simulink model "bh_proto_swingup_NEGATE_DAMPING"  (R2017a)
settings: Solver=ode4  StartTime=0.0  StopTime=11  FixedStep=0.001  RelTol=1e-5  EnableMultiTasking=on
values from neighbouring files (symbols this model uses):
  b3_damp = res_T.b3_damp    [bh_pend_solve_ODE_sys.m]
  Io3_xx = res_T.Io3_xx    [bh_pend_solve_ODE_sys.m]
  L3y = res_T.L3y    [bh_pend_solve_ODE_sys.m]    (also in bh_pend_solve_ODE_sys_custom.m)
  m = res_T.mass3    [bh_pend_solve_ODE_sys_custom.m]
  mass3 = res_T.mass3    [bh_pend_solve_ODE_sys.m]    (also in bh_pend_solve_ODE_sys_custom.m)
  N = 1 + N_steps    [bh_pend_solve_ODE_sys_custom.m]
undefined symbols (not defined in the file or in its folder): L3x, L3z, X, Y, Z
libraries: sm_lib x12, simulink_extras x11, nesl_utility x8, simulink x2
settings Model: Creator=bhorton  LastModifiedBy=bhorton
settings SolverCC: ZeroCrossAlgorithm=Adaptive
settings OptimizationCC: LifeSpan=inf
settings DebuggingCC: SFUnexpectedBacktrackingDiag=warning  SFNoUnconditionalDefaultTransitionDiag=warning  SFExecutionAtInitializationDiag=none
settings GRTTargetCC: TargetLangStandard=C89/C90 (ANSI)
settings ConfigComp: CovMetricSettings=dw  CovHtmlReporting=on  CovSaveCumulativeToWorkspaceVar=on  CovSaveSingleToWorkspaceVar=on  CovExternalEMLEnable=off
settings SimscapeCC: SimscapeLogType=all  SimscapeLogDataHistory=10000  SelectedTab=Simscape Multibody

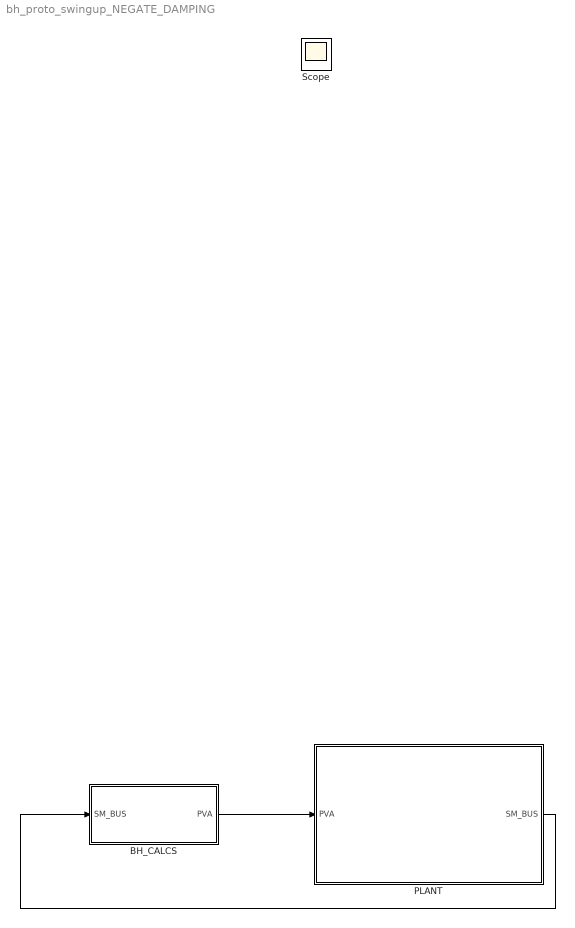
== system bh_proto_swingup_NEGATE_DAMPING ==
  BH_CALCS : Subsystem
  PLANT : Subsystem
  Scope : Scope
  wires:
  PLANT/1(SM_BUS) -> BH_CALCS/1(SM_BUS)
  BH_CALCS/1(PVA) -> PLANT/1(PVA)

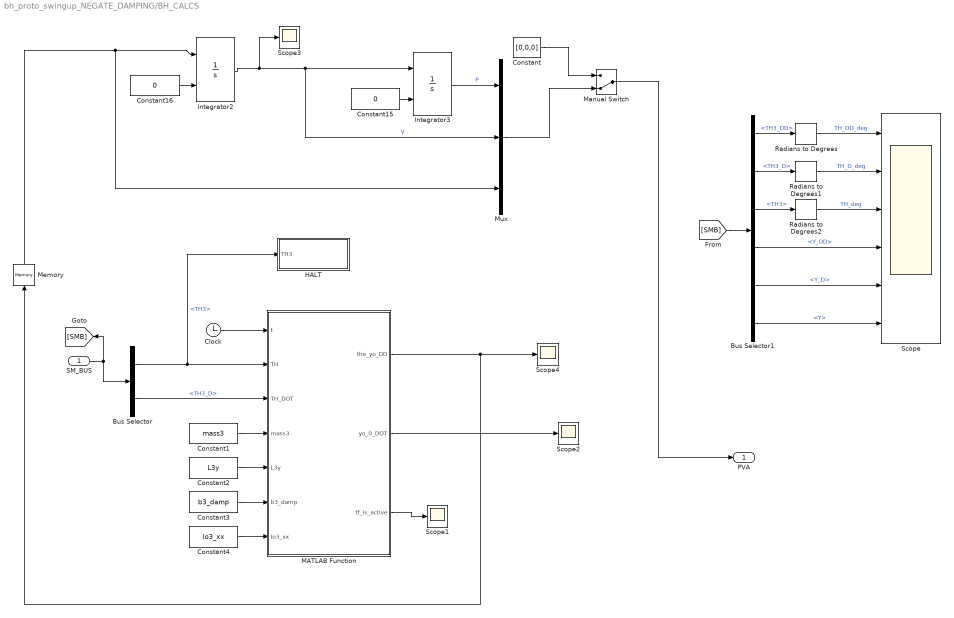
== system bh_proto_swingup_NEGATE_DAMPING/BH_CALCS ==
  SM_BUS : Inport
  Bus Selector : BusSelector  OutputSignals=TH3,TH3_D
  Bus Selector1 : BusSelector  OutputSignals=TH3_DD,TH3_D,TH3,Y_DD,Y_D,Y
  Clock : Clock
  Constant : Constant  Value=[0,0,0]
  Constant1 : Constant  Value=mass3
  Constant15 : Constant  Value=0
  Constant16 : Constant  Value=0
  Constant2 : Constant  Value=L3y
  Constant3 : Constant  Value=b3_damp
  Constant4 : Constant  Value=Io3_xx
  HALT : Subsystem
  Integrator2 : Integrator  InitialConditionSource=external
  Integrator3 : Integrator  InitialConditionSource=external
  MATLAB Function : MATLAB Function  TreatAsAtomicUnit=on  SystemSampleTime=0.001
  Manual Switch : ManualSwitch  CurrentSetting=0
  Memory : Memory
  Mux : Mux  Inputs=3
  Radians to Degrees : simulink_extras/Transformations/Radians to Degrees
  Radians to Degrees1 : simulink_extras/Transformations/Radians to Degrees
  Radians to Degrees2 : simulink_extras/Transformations/Radians to Degrees
  Scope : Scope  NumInputPorts=6
  Scope{1..4} (4 alike) : Scope
  PVA : Outport
  wires:
  Integrator3/1 -> Mux/1  "P"
  Integrator2/1 -> Scope3/1, Mux/2, Integrator3/1  "V"
  Constant15/1 -> Integrator3/2
  Manual Switch/1 -> PVA/1
  SM_BUS/1 -> [SMB], Bus Selector/1
  Bus Selector/1 -> HALT/1(TH3), MATLAB Function/2(TH)  "<TH3>"
  Bus Selector/2 -> MATLAB Function/3(TH_DOT)  "<TH3_D>"
  Memory/1 -> Mux/3, Integrator2/1
  Constant3/1 -> MATLAB Function/6(b3_damp)
  Constant2/1 -> MATLAB Function/5(L3y)
  Constant1/1 -> MATLAB Function/4(mass3)
  MATLAB Function/1(the_yo_DD) -> Scope4/1, Memory/1
  [SMB] -> Bus Selector1/1
  Bus Selector1/1 -> Radians to Degrees/1  "<TH3_DD>"
  Bus Selector1/2 -> Radians to Degrees1/1  "<TH3_D>"
  Bus Selector1/3 -> Radians to Degrees2/1  "<TH3>"
  Radians to Degrees/1 -> Scope/1  "TH_DD_deg"
  Radians to Degrees1/1 -> Scope/2  "TH_D_deg"
  Radians to Degrees2/1 -> Scope/3  "TH_deg"
  Bus Selector1/4 -> Scope/4  "<Y_DD>"
  Bus Selector1/5 -> Scope/5  "<Y_D>"
  Bus Selector1/6 -> Scope/6  "<Y>"
  Mux/1 -> Manual Switch/2
  Constant/1 -> Manual Switch/1
  Clock/1 -> MATLAB Function/1(t)
  MATLAB Function/3(tf_is_active) -> Scope1/1
  MATLAB Function/2(yo_0_DOT) -> Scope2/1
  Constant4/1 -> MATLAB Function/7(Io3_xx)
  Constant16/1 -> Integrator2/2

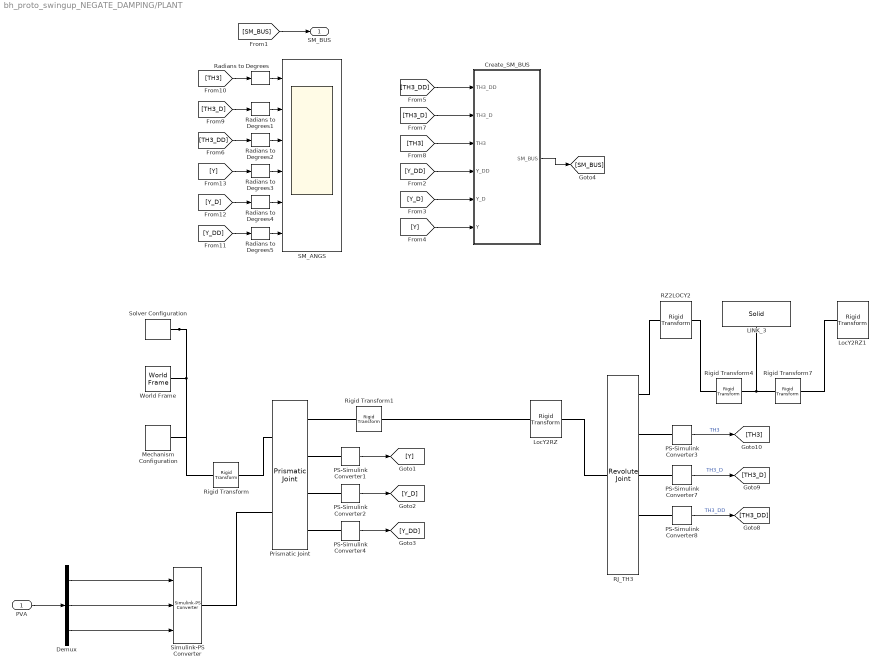
== system bh_proto_swingup_NEGATE_DAMPING/PLANT ==
  PVA : Inport
  Create_SM_BUS : Subsystem
  Demux : Demux  Outputs=3
  LINK_3 : sm_lib/Body Elements/Solid  InertiaType=CalculateFromGeometry  Mass=1  MassUnits=kg  CenterOfMass=[0 0 0]  CenterOfMassUnits=m  MomentsOfInertia=[1 1 1]  MomentsOfInertiaUnits=kg*m^2  ProductsOfInertia=[0 0 0]  ProductsOfInertiaUnits=kg*m^2  DensityBased=on  Density=density  DensityUnits=kg/(m^3)  DoExposeReferenceFrame=on  SerializedFrames=<Frames/>  GraphicType=FromGeometry  MarkerShape=Sphere  MarkerSize=10  GraphicVisPropType=SimpleVisualProperties  GraphicDiffuseColor=[1.0 0.8 0.4]  GraphicSpecularColor=[0.5 0.5 0.5 1.0]  GraphicAmbientColor=[0.15 0.15 0.15 1.0]  GraphicEmissiveColor=[0.0 0.0 0.0 1.0]  GraphicShininess=75  GraphicOpacity=1.0  GeometryShape=Brick  RectangleSize=[1 1]  RectangleSizeUnits=m  BrickDimensions=[L3x, L3y, L3z ]  BrickDimensionUnits=m  CylinderRadius=1  CylinderRadiusUnits=m  CylinderLength=1  CylinderLengthUnits=m  SphereRadius=1  SphereRadiusUnits=m  EllipsoidRadii=[1 1 1]  EllipsoidRadiiUnits=m  ExtrusionCrossSection=[1 1; -1 1; -1 -1; 1 -1]  ExtrusionCrossSectionUnits=m  ExtrusionLength=1  ExtrusionLengthUnits=m  PolygonNumSides=3  PolygonOuterRadius=1  PolygonOuterRadiusUnits=m  ExtGeomFileType=STEP  ExtGeomFileUnits=m  RevolutionCrossSection=[1 1; 1 -1; 2 -1; 2 1]  RevolutionCrossSectionUnits=m  RevolutionExtent=Full  RevolutionAngle=180  RevolutionAngleUnits=deg
  LocY2RZ : sm_lib/Frames and Transforms/Rigid Transform  TranslationMethod=None  TranslationStandardOffset=0  TranslationLengthUnit=m  TranslationStandardAxis=+Z  TranslationCartesianOffset=[0 0 0]  TranslationROffset=0  TranslationROffsetUnits=m  TranslationZOffset=0  TranslationZOffsetUnits=m  TranslationThetaOffset=0  TranslationThetaOffsetUnits=deg  RotationMethod=AlignedAxes  RotationAngleUnits=deg  RotationStandardAxis=+Z  RotationAngle=0.0  RotationArbitraryAxis=[0 0 1]  FollAlignAxisA=+X  BaseAlignAxisA=+Y  FollAlignAxisB=+Y  BaseAlignAxisB=+Z  RotationSequenceAxes=FollowerAxes  RotationSequence=XYX  RotationSequenceAngles=[0 0 0]  RotationSequenceAnglesUnits=deg  RotationMatrix=[1 0 0; 0 1 0; 0 0 1]
  LocY2RZ1 : sm_lib/Frames and Transforms/Rigid Transform  TranslationMethod=None  TranslationStandardOffset=0  TranslationLengthUnit=m  TranslationStandardAxis=+Z  TranslationCartesianOffset=[0 0 0]  TranslationROffset=0  TranslationROffsetUnits=m  TranslationZOffset=0  TranslationZOffsetUnits=m  TranslationThetaOffset=0  TranslationThetaOffsetUnits=deg  RotationMethod=AlignedAxes  RotationAngleUnits=deg  RotationStandardAxis=+Z  RotationAngle=0.0  RotationArbitraryAxis=[0 0 1]  FollAlignAxisA=+X  BaseAlignAxisA=+Y  FollAlignAxisB=+Y  BaseAlignAxisB=+Z  RotationSequenceAxes=FollowerAxes  RotationSequence=XYX  RotationSequenceAngles=[0 0 0]  RotationSequenceAnglesUnits=deg  RotationMatrix=[1 0 0; 0 1 0; 0 0 1]
  Mechanism Configuration : sm_lib/Utilities/Mechanism Configuration  UniformGravity=Constant  GravityVector=[0 0 -9.80665 ]  GravityUnits=m/s^2  LinearizationDelta=1e-4
  PS-Simulink Converter1 : nesl_utility/PS-Simulink Converter  PhysicalDomain=network_engine_domain  SubClassName=ps_output  LeftPortType=input  RightPortType=output  PseudoPeriodic=off  Frequencies=[]  Unit=m  AffineConversion=off
  PS-Simulink Converter2 : nesl_utility/PS-Simulink Converter  PhysicalDomain=network_engine_domain  SubClassName=ps_output  LeftPortType=input  RightPortType=output  PseudoPeriodic=off  Frequencies=[]  Unit=m/s  AffineConversion=off
  PS-Simulink Converter3 : nesl_utility/PS-Simulink Converter  PhysicalDomain=network_engine_domain  SubClassName=ps_output  LeftPortType=input  RightPortType=output  PseudoPeriodic=off  Frequencies=[]  Unit=rad  AffineConversion=off
  PS-Simulink Converter4 : nesl_utility/PS-Simulink Converter  PhysicalDomain=network_engine_domain  SubClassName=ps_output  LeftPortType=input  RightPortType=output  PseudoPeriodic=off  Frequencies=[]  Unit=m/s^2  AffineConversion=off
  PS-Simulink Converter7 : nesl_utility/PS-Simulink Converter  PhysicalDomain=network_engine_domain  SubClassName=ps_output  LeftPortType=input  RightPortType=output  PseudoPeriodic=off  Frequencies=[]  Unit=rad/s  AffineConversion=off
  PS-Simulink Converter8 : nesl_utility/PS-Simulink Converter  PhysicalDomain=network_engine_domain  SubClassName=ps_output  LeftPortType=input  RightPortType=output  PseudoPeriodic=off  Frequencies=[]  Unit=rad/s^2  AffineConversion=off
  Prismatic Joint : sm_lib/Joints/Prismatic Joint  SenseConstraintForce=off  SenseConstraintForceX=off  SenseConstraintForceY=off  SenseConstraintForceZ=off  SenseConstraintTorque=off  SenseConstraintTorqueX=off  SenseConstraintTorqueY=off  SenseConstraintTorqueZ=off  SenseTotalForce=off  SenseTotalForceX=off  SenseTotalForceY=off  SenseTotalForceZ=off  SenseTotalTorque=off  SenseTotalTorqueX=off  SenseTotalTorqueY=off  SenseTotalTorqueZ=off  CompositeWrenchDir=FollowerOnBase  CompositeWrenchFrame=BaseFrame  EquilibriumPosition=0  EquilibriumPositionUnits=m  SpringStiffness=0  SpringStiffnessUnits=N/m  DampingCoefficient=0  DampingCoefficientUnits=N/(m/s)  TorqueActuationMode=ComputedTorque  MotionActuationMode=InputMotion  SensePosition=on  SenseVelocity=on  SenseAcceleration=on  SenseTorqueForce=off  PositionTargetSpecify=off  PositionTargetPriority=High  PositionTargetValue=0  PositionTargetValueUnits=m  VelocityTargetSpecify=off  VelocityTargetPriority=High  VelocityTargetValue=0  VelocityTargetValueUnits=m/s
  RJ_TH3 : sm_lib/Joints/Revolute Joint  SenseConstraintForce=on  SenseConstraintForceX=off  SenseConstraintForceY=off  SenseConstraintForceZ=off  SenseConstraintTorque=off  SenseConstraintTorqueX=off  SenseConstraintTorqueY=off  SenseConstraintTorqueZ=off  SenseTotalForce=off  SenseTotalForceX=off  SenseTotalForceY=off  SenseTotalForceZ=off  SenseTotalTorque=off  SenseTotalTorqueX=off  SenseTotalTorqueY=off  SenseTotalTorqueZ=off  CompositeWrenchDir=BaseOnFollower  CompositeWrenchFrame=BaseFrame  EquilibriumPosition=0  EquilibriumPositionUnits=deg  SpringStiffness=0  SpringStiffnessUnits=N*m/deg  DampingCoefficient=b3_damp  DampingCoefficientUnits=N*m/(rad/s)  TorqueActuationMode=NoTorque  MotionActuationMode=ComputedMotion  SensePosition=on  SenseVelocity=on  SenseAcceleration=on  SenseTorqueForce=off  PositionTargetSpecify=on  PositionTargetPriority=Low  PositionTargetValue=-1  PositionTargetValueUnits=deg  VelocityTargetSpecify=on  VelocityTargetPriority=High  VelocityTargetValue=0  VelocityTargetValueUnits=rad/s
      settings: AttributesFormatString=|
      | %<DampingCoefficient>
      | %<PositionTargetValue>
      | %<VelocityTargetValue>
  RZ2LOCY2 : sm_lib/Frames and Transforms/Rigid Transform  TranslationMethod=None  TranslationStandardOffset=0  TranslationLengthUnit=m  TranslationStandardAxis=+Z  TranslationCartesianOffset=[0 0 0]  TranslationROffset=0  TranslationROffsetUnits=m  TranslationZOffset=0  TranslationZOffsetUnits=m  TranslationThetaOffset=0  TranslationThetaOffsetUnits=deg  RotationMethod=AlignedAxes  RotationAngleUnits=deg  RotationStandardAxis=+Z  RotationAngle=0.0  RotationArbitraryAxis=[0 0 1]  FollAlignAxisA=+Y  BaseAlignAxisA=+X  FollAlignAxisB=+X  BaseAlignAxisB=+Z  RotationSequenceAxes=FollowerAxes  RotationSequence=XYX  RotationSequenceAngles=[0 0 0]  RotationSequenceAnglesUnits=deg  RotationMatrix=[1 0 0; 0 1 0; 0 0 1]
  Radians to Degrees{,1..5} (6 alike) : simulink_extras/Transformations/Radians to Degrees
  Rigid Transform : sm_lib/Frames and Transforms/Rigid Transform  TranslationMethod=None  TranslationStandardOffset=0  TranslationLengthUnit=m  TranslationStandardAxis=+Z  TranslationCartesianOffset=[0 0 0]  TranslationROffset=0  TranslationROffsetUnits=m  TranslationZOffset=0  TranslationZOffsetUnits=m  TranslationThetaOffset=0  TranslationThetaOffsetUnits=deg  RotationMethod=AlignedAxes  RotationAngleUnits=deg  RotationStandardAxis=+Z  RotationAngle=0.0  RotationArbitraryAxis=[0 0 1]  FollAlignAxisA=+X  BaseAlignAxisA=+X  FollAlignAxisB=+Z  BaseAlignAxisB=+Y  RotationSequenceAxes=FollowerAxes  RotationSequence=XYX  RotationSequenceAngles=[0 0 0]  RotationSequenceAnglesUnits=deg  RotationMatrix=[1 0 0; 0 1 0; 0 0 1]
  Rigid Transform1 : sm_lib/Frames and Transforms/Rigid Transform  TranslationMethod=None  TranslationStandardOffset=0  TranslationLengthUnit=m  TranslationStandardAxis=+Z  TranslationCartesianOffset=[0 0 0]  TranslationROffset=0  TranslationROffsetUnits=m  TranslationZOffset=0  TranslationZOffsetUnits=m  TranslationThetaOffset=0  TranslationThetaOffsetUnits=deg  RotationMethod=AlignedAxes  RotationAngleUnits=deg  RotationStandardAxis=+Z  RotationAngle=0.0  RotationArbitraryAxis=[0 0 1]  FollAlignAxisA=+X  BaseAlignAxisA=+X  FollAlignAxisB=+Y  BaseAlignAxisB=+Z  RotationSequenceAxes=FollowerAxes  RotationSequence=XYX  RotationSequenceAngles=[0 0 0]  RotationSequenceAnglesUnits=deg  RotationMatrix=[1 0 0; 0 1 0; 0 0 1]
  Rigid Transform4 : sm_lib/Frames and Transforms/Rigid Transform  TranslationMethod=StandardAxis  TranslationStandardOffset=L3y/2  TranslationLengthUnit=m  TranslationStandardAxis=+Y  TranslationCartesianOffset=[0 0 0]  TranslationROffset=0  TranslationROffsetUnits=m  TranslationZOffset=0  TranslationZOffsetUnits=m  TranslationThetaOffset=0  TranslationThetaOffsetUnits=deg  RotationMethod=None  RotationAngleUnits=deg  RotationStandardAxis=+Z  RotationAngle=0.0  RotationArbitraryAxis=[0 0 1]  FollAlignAxisA=+X  BaseAlignAxisA=+Y  FollAlignAxisB=+Y  BaseAlignAxisB=+Z  RotationSequenceAxes=FollowerAxes  RotationSequence=XYX  RotationSequenceAngles=[0 0 0]  RotationSequenceAnglesUnits=deg  RotationMatrix=[1 0 0; 0 1 0; 0 0 1]
  Rigid Transform7 : sm_lib/Frames and Transforms/Rigid Transform  TranslationMethod=StandardAxis  TranslationStandardOffset=L3y/2  TranslationLengthUnit=m  TranslationStandardAxis=+Y  TranslationCartesianOffset=[0 0 0]  TranslationROffset=0  TranslationROffsetUnits=m  TranslationZOffset=0  TranslationZOffsetUnits=m  TranslationThetaOffset=0  TranslationThetaOffsetUnits=deg  RotationMethod=None  RotationAngleUnits=deg  RotationStandardAxis=+Z  RotationAngle=0.0  RotationArbitraryAxis=[0 0 1]  FollAlignAxisA=+X  BaseAlignAxisA=+Y  FollAlignAxisB=+Y  BaseAlignAxisB=+Z  RotationSequenceAxes=FollowerAxes  RotationSequence=XYX  RotationSequenceAngles=[0 0 0]  RotationSequenceAnglesUnits=deg  RotationMatrix=[1 0 0; 0 1 0; 0 0 1]
  SM_ANGS : Scope  NumInputPorts=6
  Simulink-PS Converter : nesl_utility/Simulink-PS Converter  PhysicalDomain=network_engine_domain  SubClassName=ps_input  LeftPortType=input  RightPortType=output  PseudoPeriodic=off  Frequencies=[]  NoiseDistribution=none  NoiseParameters=[]  Unit=m  AffineConversion=off  FilteringAndDerivatives=provide  SimscapeFilterOrder=1  InputFilterTimeConstant=0.001  UdotUserProvided=2
  Solver Configuration : nesl_utility/Solver Configuration  PhysicalDomain=network_engine_domain  SubClassName=solver  LeftPortType=input  RightPortType=generic  Accelerate=off  Tones=[]  Harmonics=[]  SimulateNoise=off  Profile=off  UseLocalSampling=off  EnableSwitchedLinearOptims=on  FrequencyDomain=off  UseCCode=off  RelTol=0.001  AbsTol=1e-06  MinStep=1e-09  ToWorkspace=off  RevertToSquareIcSolve=off  NumHomotopyIterations=100  PhasorMode=off  PhasorModeNumHarmonics=1  OverrideAbsTol=off  DoDC=off  ResidualTolerance=1e-09  UseLocalSolver=off  LocalSolverChoice=NE_TRAPEZOIDAL_ADVANCER  LocalSolverSampleTime=0.01  DoFixedCost=off  MaxNonlinIter=3  MaxModeIter=2  LinearAlgebra=Sparse  DelaysMemoryBudget=1024  AutomaticFiltering=off  FilteringTimeConstant=0.001
  World Frame : sm_lib/Frames and Transforms/World Frame
  SM_BUS : Outport
  wires:
  Demux/2 -> Simulink-PS Converter/2
  [TH3] -> Create_SM_BUS/3(TH3)
  [Y] -> Radians to Degrees3/1
  [Y] -> Create_SM_BUS/6(Y)
  PS-Simulink Converter7/1 -> [TH3_D]  "TH3_D"
  Demux/1 -> Simulink-PS Converter/1
  [TH3_D] -> Radians to Degrees1/1
  Create_SM_BUS/1(SM_BUS) -> [SM_BUS]
  [TH3_D] -> Create_SM_BUS/2(TH3_D)
  [TH3_DD] -> Create_SM_BUS/1(TH3_DD)
  PS-Simulink Converter3/1 -> [TH3]  "TH3"
  PS-Simulink Converter1/1 -> [Y]
  [SM_BUS] -> SM_BUS/1
  Demux/3 -> Simulink-PS Converter/3
  PVA/1 -> Demux/1
  [TH3] -> Radians to Degrees/1
  PS-Simulink Converter8/1 -> [TH3_DD]  "TH3_DD"
  PS-Simulink Converter4/1 -> [Y_DD]
  [Y_DD] -> Create_SM_BUS/4(Y_DD)
  PS-Simulink Converter2/1 -> [Y_D]
  [Y_DD] -> Radians to Degrees5/1
  [TH3_DD] -> Radians to Degrees2/1
  [Y_D] -> Create_SM_BUS/5(Y_D)
  [Y_D] -> Radians to Degrees4/1
  Radians to Degrees/1 -> SM_ANGS/1
  Radians to Degrees1/1 -> SM_ANGS/2
  Radians to Degrees2/1 -> SM_ANGS/3
  Radians to Degrees3/1 -> SM_ANGS/4
  Radians to Degrees4/1 -> SM_ANGS/5
  Radians to Degrees5/1 -> SM_ANGS/6
  connections:
  Solver Configuration/RConn1 -- World Frame/RConn1 -- Rigid Transform/LConn1 -- Mechanism Configuration/RConn1
  RZ2LOCY2/RConn1 -- Rigid Transform4/LConn1
  PS-Simulink Converter3/LConn1 -- RJ_TH3/RConn2
  Prismatic Joint/LConn1 -- Rigid Transform/RConn1
  PS-Simulink Converter4/LConn1 -- Prismatic Joint/RConn4
  LocY2RZ1/LConn1 -- Rigid Transform7/RConn1
  Prismatic Joint/RConn2 -- PS-Simulink Converter1/LConn1
  LocY2RZ/LConn1 -- Rigid Transform1/RConn1
  RJ_TH3/LConn1 -- LocY2RZ/RConn1
  Simulink-PS Converter/RConn1 -- Prismatic Joint/LConn2
  Rigid Transform4/RConn1 -- LINK_3/RConn1 -- Rigid Transform7/LConn1
  RJ_TH3/RConn3 -- PS-Simulink Converter7/LConn1
  Rigid Transform1/LConn1 -- Prismatic Joint/RConn1
  RJ_TH3/RConn4 -- PS-Simulink Converter8/LConn1
  PS-Simulink Converter2/LConn1 -- Prismatic Joint/RConn3
  RZ2LOCY2/LConn1 -- RJ_TH3/RConn1

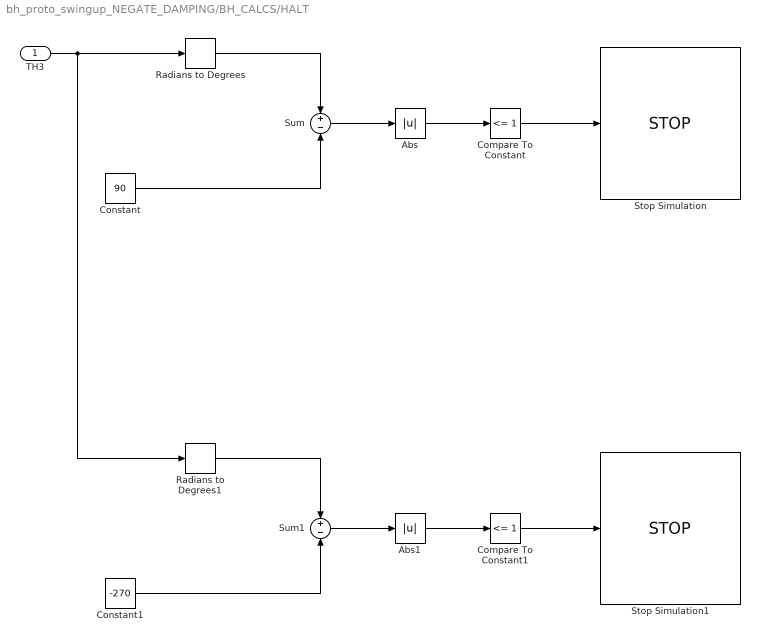
== system bh_proto_swingup_NEGATE_DAMPING/BH_CALCS/HALT ==
  TH3 : Inport
  Abs : Abs
  Abs1 : Abs
  Compare To Constant : simulink/Logic and Bit Operations/Compare To Constant  relop=<=  const=1  OutDataTypeStr=boolean
  Compare To Constant1 : simulink/Logic and Bit Operations/Compare To Constant  relop=<=  const=1  OutDataTypeStr=boolean
  Constant : Constant  Value=90
  Constant1 : Constant  Value=-270
  Radians to Degrees : simulink_extras/Transformations/Radians to Degrees
  Radians to Degrees1 : simulink_extras/Transformations/Radians to Degrees
  Stop Simulation : Stop
  Stop Simulation1 : Stop
  Sum : Sum  Inputs=+|-
  Sum1 : Sum  Inputs=+|-
  wires:
  TH3/1 -> Radians to Degrees1/1, Radians to Degrees/1
  Radians to Degrees/1 -> Sum/1
  Constant/1 -> Sum/2
  Sum/1 -> Abs/1
  Abs/1 -> Compare To Constant/1
  Compare To Constant/1 -> Stop Simulation/1
  Compare To Constant1/1 -> Stop Simulation1/1
  Sum1/1 -> Abs1/1
  Radians to Degrees1/1 -> Sum1/1
  Constant1/1 -> Sum1/2
  Abs1/1 -> Compare To Constant1/1

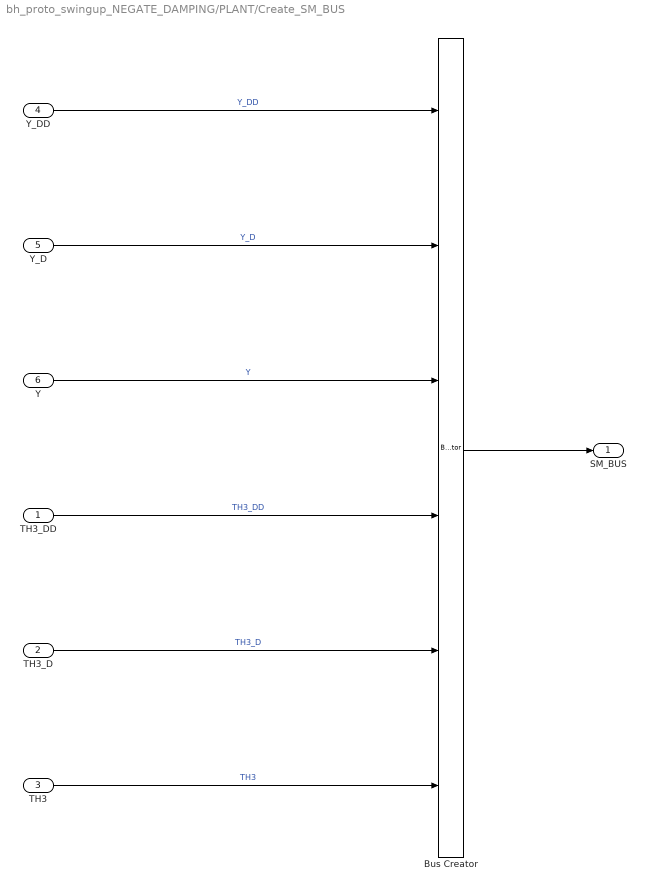
== system bh_proto_swingup_NEGATE_DAMPING/PLANT/Create_SM_BUS ==
  TH3_DD : Inport
  TH3_D : Inport  Port=2
  TH3 : Inport  Port=3
  Y_DD : Inport  Port=4
  Y_D : Inport  Port=5
  Y : Inport  Port=6
  Bus Creator : BusCreator  Inputs=6
  SM_BUS : Outport
  wires:
  Bus Creator/1 -> SM_BUS/1
  TH3/1 -> Bus Creator/6  "TH3"
  TH3_D/1 -> Bus Creator/5  "TH3_D"
  TH3_DD/1 -> Bus Creator/4  "TH3_DD"
  Y_D/1 -> Bus Creator/2  "Y_D"
  Y/1 -> Bus Creator/3  "Y"
  Y_DD/1 -> Bus Creator/1  "Y_DD"

== matlab function bh_proto_swingup_NEGATE_DAMPING/BH_CALCS/MATLAB Function ==
  data: t input; TH input; the_yo_DD output; TH_DOT input; mass3 input; L3y input; b3_damp input; yo_0_DOT output; tf_is_active output; Io3_xx input
function [the_yo_DD, yo_0_DOT, tf_is_active] = fcn(t, TH, TH_DOT, mass3, L3y, b3_damp, Io3_xx)

the_yo_DD    = 0;
yo_0_DOT     = 0;
tf_is_active = 0;

    theta     = TH;   
    theta_dot = TH_DOT;

    if( abs(theta) < 0.001 )
          THE_SIGN = sign(theta);
          if(0==THE_SIGN)
              THE_SIGN = 1;
          end
          the_yo_DD = theta_dot/(THE_SIGN*0.001);
    else
          the_yo_DD = theta_dot/sin(theta);
    end

    k          =     1.04 * b3_damp * (2/(mass3 * L3y));
    %k          =     5 * b3_damp * (2/(mass3 * L3y));
    the_yo_DD  =     k   * the_yo_DD;

%     if(abs(the_yo_DD) > 30)
%        the_yo_DD = sign(the_yo_DD) * 30;
%     end

   tf_is_active = 1;
